simulink model "ContinuosModelExam"  (R2023b)
settings: Solver=VariableStepAuto  StartTime=0.0  StopTime=0.5  MaxStep=inverter.param.timeSwitching*0.1  RelTol=1e-3
undefined symbols (not defined in the file or in its folder): contr_D, contr_Q, contr_W, inverter, mot
settings Model: Creator=zambo  LastModifiedBy=zambo

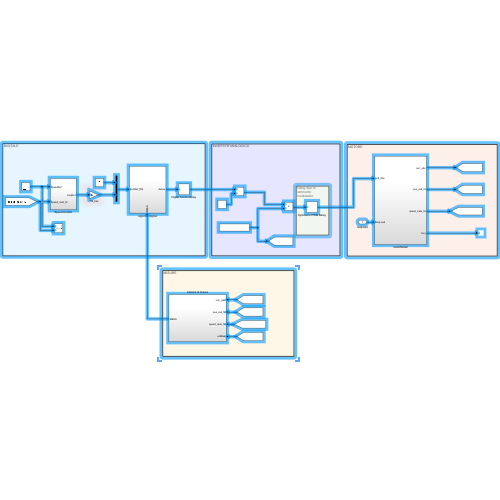
[thumbnail: Simulink's stored preview of the top-level diagram]
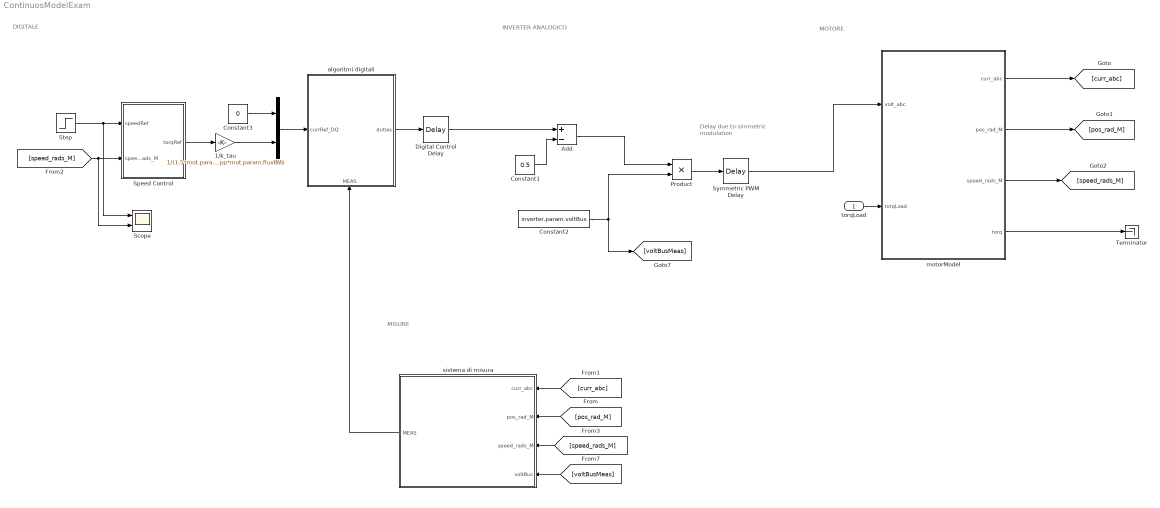
== system ContinuosModelExam ==
  note: MOTORE
  note: INVERTER ANALOGICO
  note: Delay due to
      | simmetric
      | modulation
  note: DIGITALE
  note: MISURE
  torqLoad : Inport
  1/k_tau : Gain  Gain=1/(1.5*mot.param.pp*mot.param.fluxPM)
  Add : Sum  Inputs=+-
  Constant1 : Constant  Value=0.5
  Constant2 : Constant  Value=inverter.param.voltBus
  Constant3 : Constant  Value=0
  Digital Control Delay : TransportDelay  DelayTime=inverter.param.timeSwitching
  Mux : Mux  Inputs=2
  Product : Product
  Scope : Scope  NumInputPorts=2
  Speed Control : Subsystem
  Step : Step  Time=0.2  After=290  SampleTime=0
  Symmetric PWM Delay : TransportDelay  DelayTime=inverter.param.timeSwitching*0.5
  Terminator : Terminator
  algoritmi digitali : Subsystem
      settings: PortSchema="{\"entries\":[{\"content\":{\"sides\":[{\"content\":{\"connectorIds\":[\"In1\"]},\"type\":\"ConnectorPlacement.EquallySpacedRectSide\",\"uuid\":\"be98b178-87c5-4194-8b79-c3f3cfcc0fc0\"},{\"content\":{\"connectorIds\":[\"Out1\"],\"side\":\"RIGHT\"},\"type\":\"ConnectorPlacement.EquallySpacedRectSide\",\"uuid\":\"8217c3eb-ba2e-412f-a9c4-f2e3b7cd9b00\"},{\"content\":{\"side\":\"TOP\"},\"type\":\"ConnectorPlacement.EquallySpacedRectSide\",\"uuid\":\"9b7fad55-3d61-41f3-9dee-47d3dc8a32f9\"},{\"content\":{\"connectorIds\":[\"In2\"],\"side\":\"BOTTOM\"},\"type\":\"ConnectorPlacement.EquallySpacedRectSide\",\"uuid\":\"8ebbf679-530e-4b8b-8dca-2f31264a1f1b\"}]},\"type\":\"ConnectorPlacement.EquallySpacedConnector\",\"uuid\":\"25d4c349-4b88-4de2-b9c1-687bdffd88d1\"}],\"packageUris\":[\"http://schema.mathworks.com/mf0/Connector/R2020b\"],\"version\":\"1.0\"}"
  motorModel : Subsystem
  sistema di misura : Subsystem
  wires:
  Constant3/1 -> Mux/1
  Mux/1 -> algoritmi digitali/1(currRef_DQ)
  Symmetric PWM Delay/1 -> motorModel/1(volt_abc)
  motorModel/3(speed_rads_M) -> [speed_rads_M]
  [speed_rads_M] -> Scope/2, Speed Control/2(speed_rads_M)
  Step/1 -> Scope/1, Speed Control/1(speedRef)
  Constant1/1 -> Add/2
  1/k_tau/1 -> Mux/2
  [curr_abc] -> sistema di misura/1(curr_abc)
  motorModel/2(pos_rad_M) -> [pos_rad_M]
  motorModel/4(torq) -> Terminator/1
  Speed Control/1(torqRef) -> 1/k_tau/1
  motorModel/1(curr_abc) -> [curr_abc]
  [speed_rads_M] -> sistema di misura/3(speed_rads_M)
  [voltBusMeas] -> sistema di misura/4(voltBus)
  Digital Control Delay/1 -> Add/1
  Add/1 -> Product/1
  algoritmi digitali/1(duties) -> Digital Control Delay/1
  sistema di misura/1(MEAS) -> algoritmi digitali/2(MEAS)
  [pos_rad_M] -> sistema di misura/2(pos_rad_M)
  Product/1 -> Symmetric PWM Delay/1
  Constant2/1 -> Product/2, [voltBusMeas]
  torqLoad/1 -> motorModel/2(torqLoad)

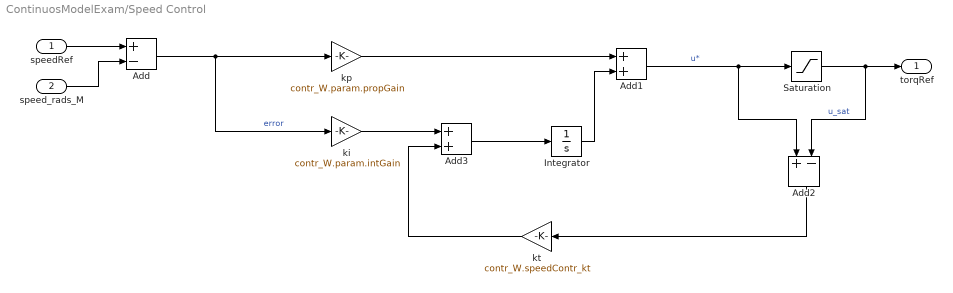
== system ContinuosModelExam/Speed Control ==
  speedRef : Inport
  speed_rads_M : Inport  Port=2
  Add : Sum  Inputs=+-
  Add1 : Sum
  Add2 : Sum  Inputs=+-
  Add3 : Sum
  Integrator : Integrator
  Saturation : Saturate  UpperLimit=0.22  LowerLimit=-0.22
  ki : Gain  Gain=contr_W.param.intGain
  kp : Gain  Gain=contr_W.param.propGain
  kt : Gain  Gain=contr_W.speedContr_kt
  torqRef : Outport
  wires:
  Integrator/1 -> Add1/2
  kp/1 -> Add1/1
  Add/1 -> ki/1, kp/1  "error"
  speedRef/1 -> Add/1
  speed_rads_M/1 -> Add/2
  Add1/1 -> Add2/1, Saturation/1  "u*"
  Saturation/1 -> Add2/2, torqRef/1  "u_sat"
  Add2/1 -> kt/1
  ki/1 -> Add3/1
  Add3/1 -> Integrator/1
  kt/1 -> Add3/2

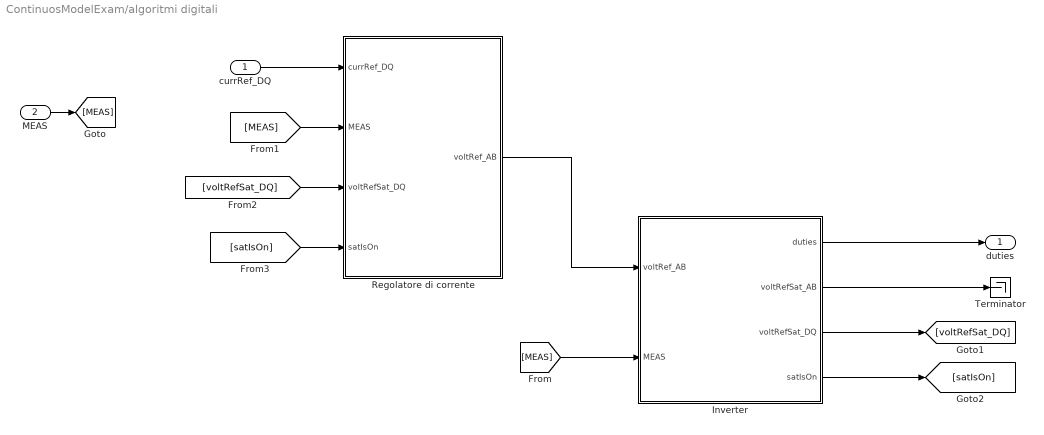
== system ContinuosModelExam/algoritmi digitali ==
  currRef_DQ : Inport
  MEAS : Inport  Port=2
  Inverter : Subsystem
  Regolatore di corrente : Subsystem
  Terminator : Terminator
  duties : Outport
  wires:
  Inverter/1(duties) -> duties/1
  MEAS/1 -> [MEAS]
  [MEAS] -> Inverter/2(MEAS)
  currRef_DQ/1 -> Regolatore di corrente/1(currRef_DQ)
  Regolatore di corrente/1(voltRef_AB) -> Inverter/1(voltRef_AB)
  Inverter/4(satIsOn) -> [satIsOn]
  [MEAS] -> Regolatore di corrente/2(MEAS)
  Inverter/3(voltRefSat_DQ) -> [voltRefSat_DQ]
  [voltRefSat_DQ] -> Regolatore di corrente/3(voltRefSat_DQ)
  [satIsOn] -> Regolatore di corrente/4(satIsOn)
  Inverter/2(voltRefSat_AB) -> Terminator/1

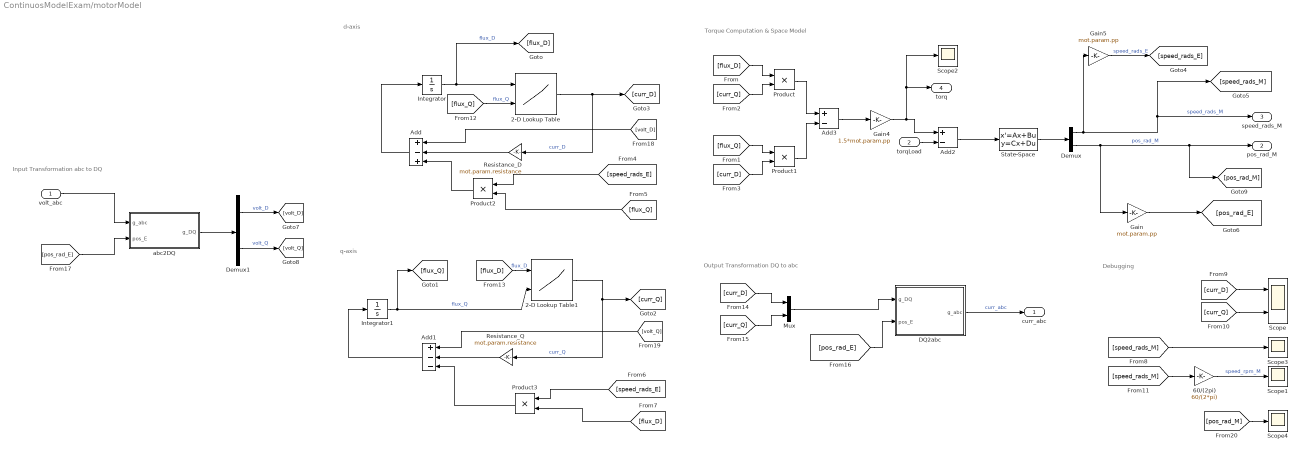
== system ContinuosModelExam/motorModel ==
  note: Debugging
  note: Torque Computation & Space Model
  note: Output Transformation DQ to abc
  note: Input Transformation abc to DQ
  note: q-axis
  note: d-axis
  volt_abc : Inport
  torqLoad : Inport  Port=2
  2-D Lookup Table : Lookup_n-D  BreakpointsForDimension1=mot.maps.fluxVec_D  BreakpointsForDimension2=mot.maps.fluxVec_Q  Table=mot.maps.currMap_D'  InternalRulePriority=Speed  RndMeth=Simplest
      settings: InputPortMap=u0,u1
  2-D Lookup Table1 : Lookup_n-D  BreakpointsForDimension1=mot.maps.fluxVec_D  BreakpointsForDimension2=mot.maps.fluxVec_Q  Table=mot.maps.currMap_Q'  InternalRulePriority=Speed  RndMeth=Simplest
      settings: InputPortMap=u0,u1
  60/(2pi) : Gain  Gain=60/(2*pi)
  Add : Sum  Inputs=+-+
  Add1 : Sum  Inputs=+--
  Add2 : Sum  Inputs=+-
  Add3 : Sum  Inputs=+-
  DQ2abc : MATLAB Function  TreatAsAtomicUnit=on
  Demux : Demux  Outputs=2
  Demux1 : Demux  Outputs=2
  Gain : Gain  Gain=mot.param.pp
  Gain4 : Gain  Gain=1.5*mot.param.pp
  Gain5 : Gain  Gain=mot.param.pp
  Integrator : Integrator  InitialCondition=mot.param.fluxPM
  Integrator1 : Integrator
  Mux : Mux  Inputs=2
  Product{,1..3} (4 alike) : Product
  Resistance_D : Gain  Gain=mot.param.resistance
  Resistance_Q : Gain  Gain=mot.param.resistance
  Scope : Scope  NumInputPorts=2
  Scope{1..4} (4 alike) : Scope
  State-Space : StateSpace  A=mot.param.Amech  B=mot.param.Bmech  C=mot.param.Cmech  D=mot.param.Dmech  InitialCondition=[0 0]
  abc2DQ : MATLAB Function  TreatAsAtomicUnit=on
  curr_abc : Outport
  pos_rad_M : Outport  Port=2
  speed_rads_M : Outport  Port=3
  torq : Outport  Port=4
  wires:
  State-Space/1 -> Demux/1
  Demux/1 -> [speed_rads_M], speed_rads_M/1, Gain5/1  "speed_rads_M"
  DQ2abc/1(g_abc) -> curr_abc/1  "curr_abc"
  2-D Lookup Table1/1 -> Resistance_Q/1, [curr_Q]  "curr_Q"
  [flux_D] -> Product/1
  [flux_Q] -> Product2/2
  [speed_rads_M] -> 60/(2pi)/1
  2-D Lookup Table/1 -> Resistance_D/1, [curr_D]  "curr_D"
  Integrator1/1 -> 2-D Lookup Table1/2, [flux_Q]  "flux_Q"
  Resistance_D/1 -> Add/2
  Resistance_Q/1 -> Add1/2
  Mux/1 -> DQ2abc/1(g_DQ)
  Gain5/1 -> [speed_rads_E]  "speed_rads_E"
  [flux_D] -> 2-D Lookup Table1/1  "flux_D"
  Gain/1 -> [pos_rad_E]
  [curr_D] -> Scope/1
  60/(2pi)/1 -> Scope1/1  "speed_rpm_M"
  [speed_rads_E] -> Product2/1
  [curr_Q] -> Scope/2
  Product1/1 -> Add3/2
  Gain4/1 -> torq/1, Scope2/1, Add2/1
  Integrator/1 -> 2-D Lookup Table/1, [flux_D]  "flux_D"
  Add3/1 -> Gain4/1
  Add/1 -> Integrator/1
  [curr_D] -> Product1/2
  Product2/1 -> Add/3
  [curr_Q] -> Product/2
  Add2/1 -> State-Space/1
  Demux/2 -> Gain/1, [pos_rad_M], pos_rad_M/1  "pos_rad_M"
  [flux_Q] -> Product1/1
  torqLoad/1 -> Add2/2
  Add1/1 -> Integrator1/1
  Product/1 -> Add3/1
  [pos_rad_E] -> DQ2abc/2(pos_E)
  Product3/1 -> Add1/3
  [speed_rads_E] -> Product3/1
  [flux_D] -> Product3/2
  [flux_Q] -> 2-D Lookup Table/2  "flux_Q"
  [curr_D] -> Mux/1
  [curr_Q] -> Mux/2
  volt_abc/1 -> abc2DQ/1(g_abc)
  [pos_rad_E] -> abc2DQ/2(pos_E)
  abc2DQ/1(g_DQ) -> Demux1/1
  Demux1/1 -> [volt_D]  "volt_D"
  Demux1/2 -> [volt_Q]  "volt_Q"
  [speed_rads_M] -> Scope3/1
  [pos_rad_M] -> Scope4/1
  [volt_D] -> Add/1
  [volt_Q] -> Add1/1

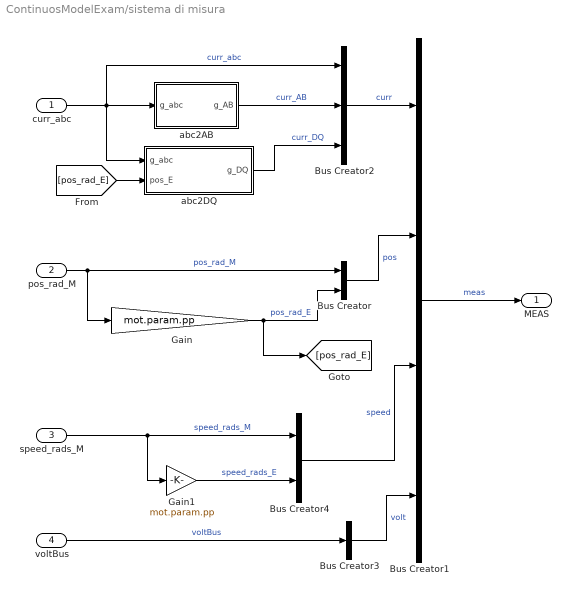
== system ContinuosModelExam/sistema di misura ==
  curr_abc : Inport
  pos_rad_M : Inport  Port=2
  speed_rads_M : Inport  Port=3
  voltBus : Inport  Port=4
  Bus Creator : BusCreator  Inputs=2
  Bus Creator1 : BusCreator  Inputs=4
  Bus Creator2 : BusCreator  Inputs=3
  Bus Creator3 : BusCreator  Inputs=1
  Bus Creator4 : BusCreator  Inputs=2
  Gain : Gain  Gain=mot.param.pp
  Gain1 : Gain  Gain=mot.param.pp
  abc2AB : MATLAB Function  TreatAsAtomicUnit=on
  abc2DQ : MATLAB Function  TreatAsAtomicUnit=on
  MEAS : Outport
  wires:
  pos_rad_M/1 -> Bus Creator/1, Gain/1  "pos_rad_M"
  Gain/1 -> [pos_rad_E], Bus Creator/2  "pos_rad_E"
  Bus Creator/1 -> Bus Creator1/2  "pos"
  curr_abc/1 -> abc2DQ/1(g_abc), Bus Creator2/1, abc2AB/1(g_abc)  "curr_abc"
  Bus Creator2/1 -> Bus Creator1/1  "curr"
  abc2DQ/1(g_DQ) -> Bus Creator2/3  "curr_DQ"
  Bus Creator1/1 -> MEAS/1  "meas"
  voltBus/1 -> Bus Creator3/1  "voltBus"
  abc2AB/1(g_AB) -> Bus Creator2/2  "curr_AB"
  [pos_rad_E] -> abc2DQ/2(pos_E)
  Bus Creator3/1 -> Bus Creator1/4  "volt"
  speed_rads_M/1 -> Gain1/1, Bus Creator4/1  "speed_rads_M"
  Gain1/1 -> Bus Creator4/2  "speed_rads_E"
  Bus Creator4/1 -> Bus Creator1/3  "speed"

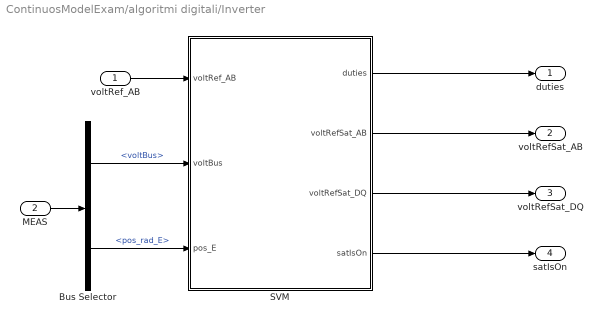
== system ContinuosModelExam/algoritmi digitali/Inverter ==
  voltRef_AB : Inport
  MEAS : Inport  Port=2
  Bus Selector : BusSelector  OutputSignals=volt.voltBus,pos.pos_rad_E
  SVM : MATLAB Function  TreatAsAtomicUnit=on
  duties : Outport
  voltRefSat_AB : Outport  Port=2
  voltRefSat_DQ : Outport  Port=3
  satIsOn : Outport  Port=4
  wires:
  SVM/4(satIsOn) -> satIsOn/1
  MEAS/1 -> Bus Selector/1
  Bus Selector/1 -> SVM/2(voltBus)  "<voltBus>"
  Bus Selector/2 -> SVM/3(pos_E)  "<pos_rad_E>"
  SVM/2(voltRefSat_AB) -> voltRefSat_AB/1
  voltRef_AB/1 -> SVM/1(voltRef_AB)
  SVM/1(duties) -> duties/1
  SVM/3(voltRefSat_DQ) -> voltRefSat_DQ/1

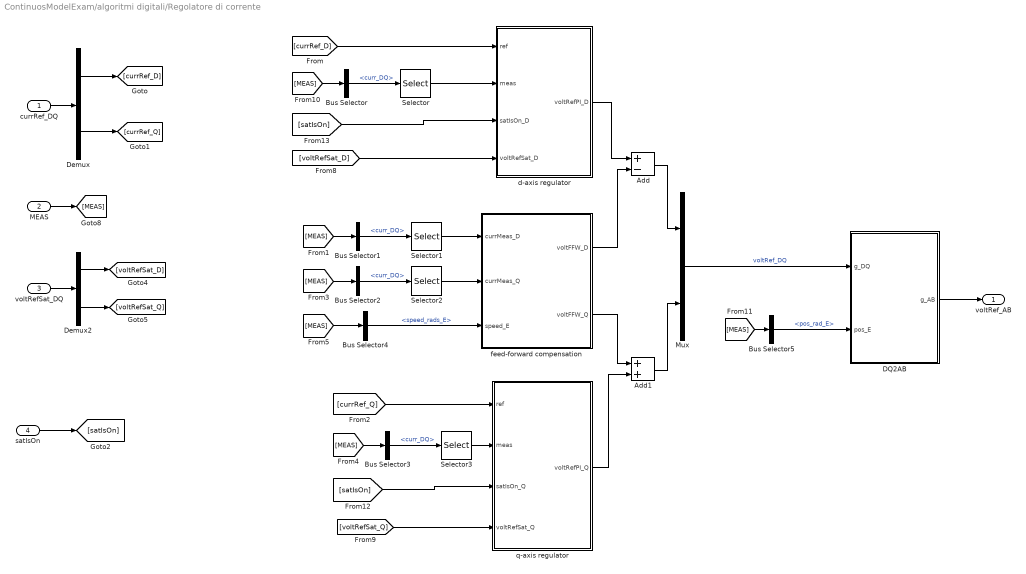
== system ContinuosModelExam/algoritmi digitali/Regolatore di corrente ==
  currRef_DQ : Inport
  MEAS : Inport  Port=2
  voltRefSat_DQ : Inport  Port=3
  satIsOn : Inport  Port=4
  Add : Sum  Inputs=+-
  Add1 : Sum
  Bus Selector{,1..3} (4 alike) : BusSelector  OutputSignals=curr.curr_DQ
  Bus Selector4 : BusSelector  OutputSignals=speed.speed_rads_E
  Bus Selector5 : BusSelector  OutputSignals=pos.pos_rad_E
  DQ2AB : MATLAB Function  TreatAsAtomicUnit=on
  Demux : Demux  Outputs=2
  Demux2 : Demux  Outputs=2
  Mux : Mux  Inputs=2
  Selector : Selector  InputPortWidth=2  IndexOptions=Index vector (dialog)  Indices=[1]  OutputSizes=1
  Selector1 : Selector  InputPortWidth=2  IndexOptions=Index vector (dialog)  Indices=[1]  OutputSizes=1
  Selector2 : Selector  InputPortWidth=2  IndexOptions=Index vector (dialog)  Indices=[2]  OutputSizes=1
  Selector3 : Selector  InputPortWidth=2  IndexOptions=Index vector (dialog)  Indices=[2]  OutputSizes=1
  d-axis regulator : Subsystem
  feed-forward compensation : Subsystem
  q-axis regulator : Subsystem
  voltRef_AB : Outport
  wires:
  currRef_DQ/1 -> Demux/1
  voltRefSat_DQ/1 -> Demux2/1
  Demux/1 -> [currRef_D]
  Demux/2 -> [currRef_Q]
  [currRef_D] -> d-axis regulator/1(ref)
  [currRef_Q] -> q-axis regulator/1(ref)
  d-axis regulator/1(voltRefPI_D) -> Add/1
  feed-forward compensation/1(voltFFW_D) -> Add/2
  feed-forward compensation/2(voltFFW_Q) -> Add1/1
  q-axis regulator/1(voltRefPI_Q) -> Add1/2
  Add1/1 -> Mux/2
  Add/1 -> Mux/1
  Demux2/1 -> [voltRefSat_D]
  Demux2/2 -> [voltRefSat_Q]
  [voltRefSat_D] -> d-axis regulator/4(voltRefSat_D)
  [voltRefSat_Q] -> q-axis regulator/4(voltRefSat_Q)
  Mux/1 -> DQ2AB/1(g_DQ)  "voltRef_DQ"
  DQ2AB/1(g_AB) -> voltRef_AB/1
  MEAS/1 -> [MEAS]
  [MEAS] -> Bus Selector/1
  Bus Selector/1 -> Selector/1  "<curr_DQ>"
  Selector/1 -> d-axis regulator/2(meas)
  Bus Selector1/1 -> Selector1/1  "<curr_DQ>"
  [MEAS] -> Bus Selector1/1
  Selector1/1 -> feed-forward compensation/1(currMeas_D)
  [MEAS] -> Bus Selector2/1
  Bus Selector2/1 -> Selector2/1  "<curr_DQ>"
  Selector2/1 -> feed-forward compensation/2(currMeas_Q)
  Bus Selector3/1 -> Selector3/1  "<curr_DQ>"
  [MEAS] -> Bus Selector3/1
  Selector3/1 -> q-axis regulator/2(meas)
  [MEAS] -> Bus Selector4/1
  Bus Selector4/1 -> feed-forward compensation/3(speed_E)  "<speed_rads_E>"
  [MEAS] -> Bus Selector5/1
  Bus Selector5/1 -> DQ2AB/2(pos_E)  "<pos_rad_E>"
  satIsOn/1 -> [satIsOn]
  [satIsOn] -> q-axis regulator/3(satIsOn_Q)
  [satIsOn] -> d-axis regulator/3(satIsOn_D)

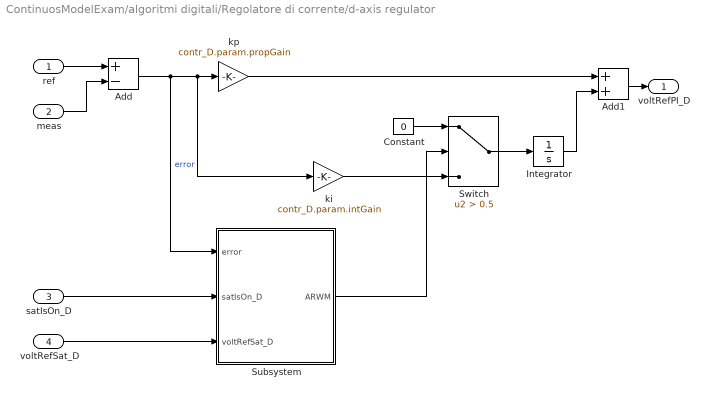
== system ContinuosModelExam/algoritmi digitali/Regolatore di corrente/d-axis regulator ==
  ref : Inport
  meas : Inport  Port=2
  satIsOn_D : Inport  Port=3
  voltRefSat_D : Inport  Port=4
  Add : Sum  Inputs=+-
  Add1 : Sum
  Constant : Constant  Value=0
  Integrator : Integrator
  Subsystem : Subsystem
  Switch : Switch  Criteria=u2 > Threshold  Threshold=0.5  SaturateOnIntegerOverflow=off  InputSameDT=off
  ki : Gain  Gain=contr_D.param.intGain
  kp : Gain  Gain=contr_D.param.propGain
  voltRefPI_D : Outport
  wires:
  meas/1 -> Add/2
  ref/1 -> Add/1
  Add/1 -> Subsystem/1(error), ki/1, kp/1  "error"
  kp/1 -> Add1/1
  Add1/1 -> voltRefPI_D/1
  Switch/1 -> Integrator/1
  Integrator/1 -> Add1/2
  Constant/1 -> Switch/1
  ki/1 -> Switch/3
  voltRefSat_D/1 -> Subsystem/3(voltRefSat_D)
  satIsOn_D/1 -> Subsystem/2(satIsOn_D)
  Subsystem/1(ARWM) -> Switch/2

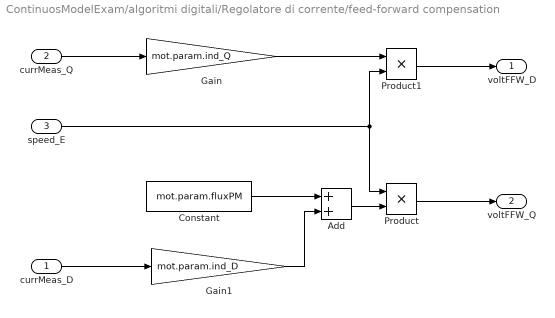
== system ContinuosModelExam/algoritmi digitali/Regolatore di corrente/feed-forward compensation ==
  currMeas_D : Inport
  currMeas_Q : Inport  Port=2
  speed_E : Inport  Port=3
  Add : Sum
  Constant : Constant  Value=mot.param.fluxPM
  Gain : Gain  Gain=mot.param.ind_Q
  Gain1 : Gain  Gain=mot.param.ind_D
  Product : Product
  Product1 : Product
  voltFFW_D : Outport
  voltFFW_Q : Outport  Port=2
  wires:
  currMeas_D/1 -> Gain1/1
  currMeas_Q/1 -> Gain/1
  Constant/1 -> Add/1
  Gain1/1 -> Add/2
  Add/1 -> Product/2
  speed_E/1 -> Product/1, Product1/2
  Gain/1 -> Product1/1
  Product1/1 -> voltFFW_D/1
  Product/1 -> voltFFW_Q/1

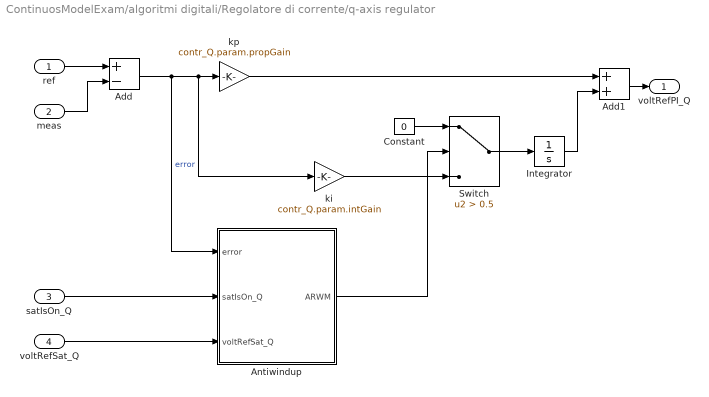
== system ContinuosModelExam/algoritmi digitali/Regolatore di corrente/q-axis regulator ==
  ref : Inport
  meas : Inport  Port=2
  satIsOn_Q : Inport  Port=3
  voltRefSat_Q : Inport  Port=4
  Add : Sum  Inputs=+-
  Add1 : Sum
  Antiwindup : Subsystem
  Constant : Constant  Value=0
  Integrator : Integrator
  Switch : Switch  Criteria=u2 > Threshold  Threshold=0.5  SaturateOnIntegerOverflow=off  InputSameDT=off
  ki : Gain  Gain=contr_Q.param.intGain
  kp : Gain  Gain=contr_Q.param.propGain
  voltRefPI_Q : Outport
  wires:
  voltRefSat_Q/1 -> Antiwindup/3(voltRefSat_Q)
  Add1/1 -> voltRefPI_Q/1
  Integrator/1 -> Add1/2
  ref/1 -> Add/1
  Switch/1 -> Integrator/1
  kp/1 -> Add1/1
  Add/1 -> Antiwindup/1(error), ki/1, kp/1  "error"
  satIsOn_Q/1 -> Antiwindup/2(satIsOn_Q)
  ki/1 -> Switch/3
  Constant/1 -> Switch/1
  Antiwindup/1(ARWM) -> Switch/2
  meas/1 -> Add/2

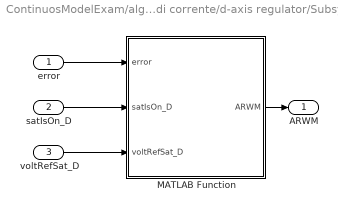
== system ContinuosModelExam/algoritmi digitali/Regolatore di corrente/d-axis regulator/Subsystem ==
  error : Inport
  satIsOn_D : Inport  Port=2
  voltRefSat_D : Inport  Port=3
  MATLAB Function : MATLAB Function  TreatAsAtomicUnit=on
  ARWM : Outport
  wires:
  satIsOn_D/1 -> MATLAB Function/2(satIsOn_D)
  error/1 -> MATLAB Function/1(error)
  voltRefSat_D/1 -> MATLAB Function/3(voltRefSat_D)
  MATLAB Function/1(ARWM) -> ARWM/1

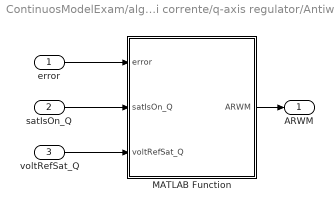
== system ContinuosModelExam/algoritmi digitali/Regolatore di corrente/q-axis regulator/Antiwindup ==
  error : Inport
  satIsOn_Q : Inport  Port=2
  voltRefSat_Q : Inport  Port=3
  MATLAB Function : MATLAB Function  TreatAsAtomicUnit=on
  ARWM : Outport
  wires:
  error/1 -> MATLAB Function/1(error)
  satIsOn_Q/1 -> MATLAB Function/2(satIsOn_Q)
  voltRefSat_Q/1 -> MATLAB Function/3(voltRefSat_Q)
  MATLAB Function/1(ARWM) -> ARWM/1

== matlab function ContinuosModelExam/algoritmi digitali/Inverter/SVM ==
  data: voltRef_AB input; voltBus input; pos_E input; duties output; voltRefSat_AB output; voltRefSat_DQ output; satIsOn output; inverter parameter
function [duties, voltRefSat_AB, voltRefSat_DQ, satIsOn] = fcn(voltRef_AB, voltBus,pos_E, inverter)

% initialize variables 
duties=ones(3,1)*0.5;
voltRefSat_AB=zeros(2,1);
satIsOn=0;

k=1;    % costante per calcolare voltRefSat_AB nel caso di saturazione circolare
k1=1;   % costante per ridurre Tm e Tm1 nel caso di saturazione esagonale
m=0;
Tm=0;
Tm1=0;
T0=0;

% define constant
c=1/sqrt(3);


% if cascade to find m
if voltRef_AB(2,1)>0.0
    if abs(voltRef_AB(1,1))>abs(voltRef_AB(2,1)*c)
        if voltRef_AB(1,1)>0.0
            m=1;
        else
            m=3;
        end
    else
        m=2;
    end
else
    if abs(voltRef_AB(1,1))>abs(voltRef_AB(2,1)*c)
        if voltRef_AB(1,1)>0.0
            m=6;
        else
            m=4;
        end
    else
        m=5;
    end
end

% Define another constant
c1=sqrt(3)*inverter.param.timeSwitching;

% circle saturation
if (inverter.param.satCircleOn==1)
    if (voltRef_AB(1,1)^2+voltRef_AB(2,1)^2)>((voltBus*c)^2)
        satIsOn=1;
        k=(voltBus*c)/(sqrt(voltRef_AB(1,1)^2+voltRef_AB(2,1)^2));
        voltRefSat_AB=k*voltRef_AB;
    end
end

% check voltBus value
if (voltBus > 0.2)
    if (satIsOn==1)
        Tm=(c1/voltBus)*(voltRefSat_AB(1,1)*sin(m*(pi/3))-voltRefSat_AB(2,1)*cos(m*(pi/3)));
        Tm1=(c1/voltBus)*(-voltRefSat_AB(1,1)*sin((m-1)*(pi/3))+voltRefSat_AB(2,1)*cos((m-1)*(pi/3)));
        T0=inverter.param.timeSwitching-Tm-Tm1;
    else
        Tm=(c1/voltBus)*(voltRef_AB(1,1)*sin(m*(pi/3))-voltRef_AB(2,1)*cos(m*(pi/3)));
        Tm1=(c1/voltBus)*(-voltRef_AB(1,1)*sin((m-1)*(pi/3))+voltRef_AB(2,1)*cos((m-1)*(pi/3)));
        T0=inverter.param.timeSwitching-Tm-Tm1;
    end
end

% hexagon saturation
if (Tm+Tm1 > inverter.param.timeSwitching)
    satIsOn=1;
    k1=inverter.param.timeSwitching/(Tm+Tm1);
    Tm=k1*Tm;
    Tm1=k1*Tm1;
    T0=0;
    voltRefSat_AB=k1*voltRef_AB;
end

% calculate duty-cycle

switch m
    case 1
        duties(1,1)=(Tm+Tm1+T0/2)*inverter.param.freqSwitching;
        duties(2,1)=(Tm1+T0/2)*inverter.param.freqSwitching;
        duties(3,1)=(T0/2)*inverter.param.freqSwitching;
    case 2
        duties(1,1)=(Tm+T0/2)*inverter.param.freqSwitching;
        duties(2,1)=(Tm+Tm1+T0/2)*inverter.param.freqSwitching;
        duties(3,1)=(T0/2)*inverter.param.freqSwitching;
    case 3
        duties(1,1)=(T0/2)*inverter.param.freqSwitching;
        duties(2,1)=(Tm+Tm1+T0/2)*inverter.param.freqSwitching;
        duties(3,1)=(Tm1+T0/2)*inverter.param.freqSwitching;
    case 4
        duties(1,1)=(T0/2)*inverter.param.freqSwitching;
        duties(2,1)=(Tm+T0/2)*inverter.param.freqSwitching;
        duties(3,1)=(Tm+Tm1+T0/2)*inverter.param.freqSwitching;
    case 5
        duties(1,1)=(Tm1+T0/2)*inverter.param.freqSwitching;
        duties(2,1)=(T0/2)*inverter.param.freqSwitching;
        duties(3,1)=(Tm+Tm1+T0/2)*inverter.param.freqSwitching;
    case 6
        duties(1,1)=(Tm+Tm1+T0/2)*inverter.param.freqSwitching;
        duties(2,1)=(T0/2)*inverter.param.freqSwitching;
        duties(3,1)=(Tm+T0/2)*inverter.param.freqSwitching;
    otherwise
        duties(1,1)=0.5;
        duties(2,1)=0.5;
        duties(3,1)=0.5;
end

% transformation from AB to DQ
voltRefSat_DQ = AB2DQ(voltRefSat_AB, pos_E);

end

== matlab function ContinuosModelExam/motorModel/DQ2abc ==
  data: g_DQ input; g_abc output; pos_E input
function g_abc = fcn(g_DQ,pos_E)

g_abc   = DQ2abc(g_DQ,pos_E);

end

== matlab function ContinuosModelExam/motorModel/abc2DQ ==
  data: g_abc input; g_DQ output; pos_E input
function g_DQ = fcn(g_abc, pos_E)

g_DQ    = abc2DQ(g_abc, pos_E);

end

== matlab function ContinuosModelExam/algoritmi digitali/Regolatore di corrente/d-axis regulator/Subsystem/MATLAB Function ==
  data: error input; ARWM output; satIsOn_D input; voltRefSat_D input
function ARWM = fcn(error, satIsOn_D, voltRefSat_D)

if ((satIsOn_D == 1) && (((voltRefSat_D < 0) && (error > 0)) || ((voltRefSat_D > 0) && (error < 0))))

    ARWM=1;

else

    ARWM=0;

end

end

== matlab function ContinuosModelExam/sistema di misura/abc2AB ==
  data: g_abc input; g_AB output
function g_AB = fcn(g_abc)

g_AB    = abc2AB(g_abc);

end

== matlab function ContinuosModelExam/sistema di misura/abc2DQ ==
  data: g_abc input; g_DQ output; pos_E input
function g_DQ = fcn(g_abc, pos_E)

g_DQ    = abc2DQ(g_abc, pos_E);

end

== matlab function ContinuosModelExam/algoritmi digitali/Regolatore di corrente/q-axis regulator/Antiwindup/MATLAB Function ==
  data: error input; ARWM output; satIsOn_Q input; voltRefSat_Q input
function ARWM = fcn(error, satIsOn_Q, voltRefSat_Q)

if ((satIsOn_Q == 1) && (((voltRefSat_Q < 0) && (error > 0)) || ((voltRefSat_Q > 0) && (error < 0))))

    ARWM=1;

else

    ARWM=0;

end

end

== matlab function ContinuosModelExam/algoritmi digitali/Regolatore di corrente/DQ2AB ==
  data: g_DQ input; g_AB output; pos_E input
function g_AB = fcn(g_DQ,pos_E)

g_AB   = DQ2AB(g_DQ,pos_E);

end
